simulink model "AutomaticLabeler"  (R2025b)
settings: Solver=VariableStepAuto  StartTime=0.0  StopTime=10.0  RelTol=1e-3
settings Model: Creator=Liam  LastModifiedBy=Liam

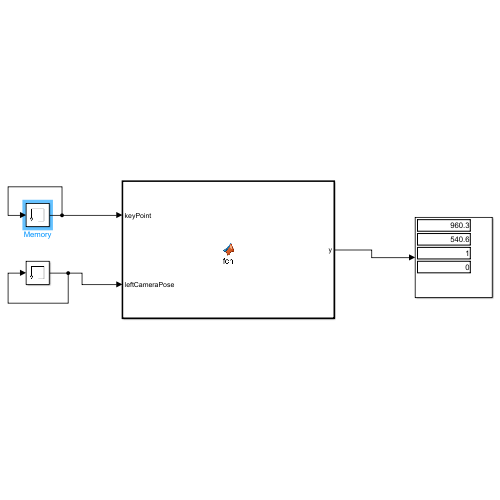
[thumbnail: Simulink's stored preview of the top-level diagram]
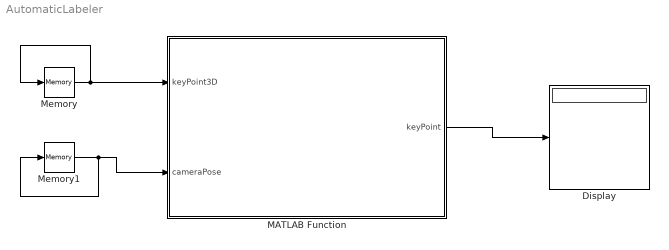
== system AutomaticLabeler ==
  Display : Display
  MATLAB Function : MATLAB Function  TreatAsAtomicUnit=on
  Memory : Memory  InitialCondition=[100 100 500]
  Memory1 : Memory  InitialCondition=[100 100 100 0 0 0]
  wires:
  Memory/1 -> Memory/1, MATLAB Function/1(keyPoint3D)
  MATLAB Function/1(keyPoint) -> Display/1
  Memory1/1 -> Memory1/1, MATLAB Function/2(cameraPose)

== matlab function AutomaticLabeler/MATLAB Function ==
  data: keyPoint output; keyPoint3D input; cameraPose input; K parameter
function keyPoint = fcn(keyPoint3D, cameraPose, K)
p = zeros(1,4);
p(1:3) = keyPoint3D(1:3);
p(4) = 1;
keyPoint = getWorldToImage(p, cameraPose, K);
